simulink model "ForEach5"  (R2017b)
settings: Solver=FixedStepDiscrete  StartTime=0.0  StopTime=10.0  FixedStep=0.200000  RelTol=1e-3  EnableMultiTasking=on
settings Model: Creator=hbourbou  LastModifiedBy=hbourbou
settings DataIOCC: LimitDataPoints=on  SaveFormat=Structure
settings OptimizationCC: LifeSpan=inf
settings DebuggingCC: SFUnexpectedBacktrackingDiag=warning  SFNoUnconditionalDefaultTransitionDiag=warning  SFExecutionAtInitializationDiag=none
settings HardwareCC: ProdBitPerPointer=32  ProdBitPerSizeT=32  ProdBitPerPtrDiffT=32  ProdLargestAtomicFloat=None  ProdIntDivRoundTo=Undefined  ProdEndianess=Unspecified  ProdWordSize=32  ProdHWDeviceType=32-bit Generic
settings ModelReferenceCC: PropagateSignalLabelsOutOfModel=off
settings CodeAppCC: StateflowObjectComments=on
settings GRTTargetCC: TargetLangStandard=C89/C90 (ANSI)  GeneratePreprocessorConditionals=Disable all
settings ConfigComp: CovMetricSettings=dw  CovHtmlReporting=on  CovSaveCumulativeToWorkspaceVar=on  CovSaveSingleToWorkspaceVar=on  CovExternalEMLEnable=off

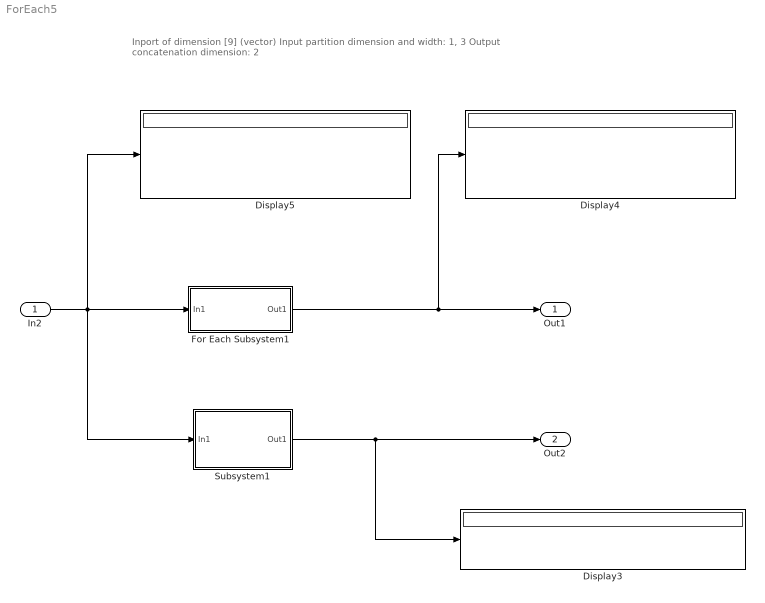
== system ForEach5 ==
  note: Inport of dimension [9] (vector)
      | Input partition dimension and width: 1, 3
      | Output concatenation dimension: 2
  In2 : Inport  PortDimensions=9
  Display3 : Display
  Display4 : Display
  Display5 : Display
  For Each Subsystem1 : Subsystem
  Subsystem1 : Subsystem
  Out1 : Outport
  Out2 : Outport  Port=2
  wires:
  In2/1 -> For Each Subsystem1/1(In1), Subsystem1/1(In1), Display5/1
  For Each Subsystem1/1(Out1) -> Out1/1, Display4/1
  Subsystem1/1(Out1) -> Out2/1, Display3/1

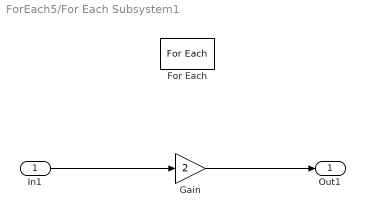
== system ForEach5/For Each Subsystem1 ==
  In1 : Inport  Partition=on  PartitionDimension=1  PartitionWidth=3  PartitionOffset=0
  For Each : ForEach  DisableCoverage=on  IndexMode=One-based
  Gain : Gain  Gain=2
  Out1 : Outport  ConcatenationDimension=2
  wires:
  Gain/1 -> Out1/1
  In1/1 -> Gain/1

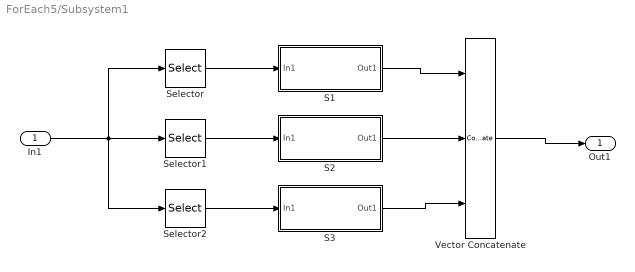
== system ForEach5/Subsystem1 ==
  In1 : Inport
  S1 : Subsystem
  S2 : Subsystem
  S3 : Subsystem
  Selector : Selector  NumberOfDimensions=2  InputPortWidth=3  IndexOptions=Index vector (dialog),Select all  Indices=[1 2 3],1  OutputSizes=1,1
  Selector1 : Selector  NumberOfDimensions=2  InputPortWidth=3  IndexOptions=Index vector (dialog),Select all  Indices=[4 5 6],1  OutputSizes=1,1
  Selector2 : Selector  NumberOfDimensions=2  InputPortWidth=3  IndexOptions=Index vector (dialog),Select all  Indices=[7 8 9],1  OutputSizes=1,1
  Vector Concatenate : Concatenate  NumInputs=3  Mode=Multidimensional array  ConcatenateDimension=2
  Out1 : Outport
  wires:
  S1/1(Out1) -> Vector Concatenate/1
  S3/1(Out1) -> Vector Concatenate/3
  S2/1(Out1) -> Vector Concatenate/2
  Selector/1 -> S1/1(In1)
  Vector Concatenate/1 -> Out1/1
  Selector2/1 -> S3/1(In1)
  Selector1/1 -> S2/1(In1)
  In1/1 -> Selector2/1, Selector1/1, Selector/1

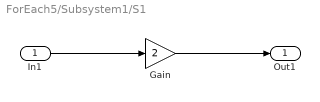
== system ForEach5/Subsystem1/S1 ==
  In1 : Inport
  Gain : Gain  Gain=2
  Out1 : Outport
  wires:
  In1/1 -> Gain/1
  Gain/1 -> Out1/1

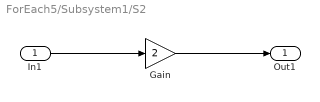
== system ForEach5/Subsystem1/S2 ==
  In1 : Inport
  Gain : Gain  Gain=2
  Out1 : Outport
  wires:
  In1/1 -> Gain/1
  Gain/1 -> Out1/1

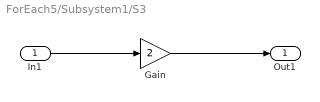
== system ForEach5/Subsystem1/S3 ==
  In1 : Inport
  Gain : Gain  Gain=2
  Out1 : Outport
  wires:
  In1/1 -> Gain/1
  Gain/1 -> Out1/1
